simulink model "BuscreaterBusselector"  (R2014a)
settings: Solver=FixedStepDiscrete  StartTime=0.0  StopTime=10.0  FixedStep=0.1  RelTol=1e-3
settings Model: CovSFcnEnable=on  BufferReuse=off  Creator=yamasefu  LastModifiedBy=ts1413
settings OptimizationCC: BlockReduction=off  OptimizeBlockIOStorage=off  BufferReuse=off  GlobalBufferReuse=off  ExpressionFolding=off  LocalBlockOutputs=off  OptimizeModelRefInitCode=on  LifeSpan=1  SimCompilerOptimization=off
settings DebuggingCC: MergeDetectMultiDrivingBlocksExec=error  SolverPrmCheckMsg=none  FrameProcessingCompatibilityMsg=error
settings RTWCC: SystemTargetFile=ert.tlc  GenCodeOnly=on  TemplateMakefile=ert_default_tmf  Description=Embedded Coder  RTWCompilerOptimization=off
settings CodeAppCC: IgnoreCustomStorageClasses=off
settings ERTTargetCC: ParMdlRefBuildCompliant=on  CompOptLevelCompliant=on  ConcurrentExecutionCompliant=on  ERTFirstTimeCompliant=on  ModelStepFunctionPrototypeControlCompliant=on  CPPClassGenCompliant=on  InlinedParameterPlacement=Hierarchical  ERTCustomFileTemplate=example_file_process.tlc

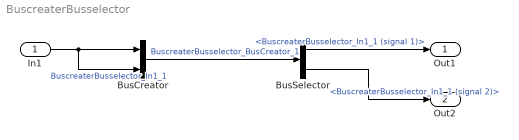
== system BuscreaterBusselector ==
  In1 : Inport
  BusCreator : BusCreator  Inputs=2
  BusSelector : BusSelector  OutputSignals=BuscreaterBusselector_In1_1 (signal 1),BuscreaterBusselector_In1_1 (signal 2)
  Out1 : Outport
  Out2 : Outport  Port=2
  wires:
  BusSelector/1 -> Out1/1  "<BuscreaterBusselector_In1_1 (signal 1)>"
  In1/1 -> BusCreator/2, BusCreator/1  "BuscreaterBusselector_In1_1"
  BusSelector/2 -> Out2/1  "<BuscreaterBusselector_In1_1 (signal 2)>"
  BusCreator/1 -> BusSelector/1  "BuscreaterBusselector_BusCreator_1"
